simulink model "ConsoleSensor_harness"  (Simulink 7.7)
settings: Solver=FixedStepDiscrete  SolverMode=SingleTasking  StartTime=0.0  StopTime=100  FixedStep=0.01  RelTol=1e-3
InitFcn:
  | if signalbuilder('ConsoleSensor_harness/Signal_Builder','activegroup') == 4
  |   CD_CONSOLE_FUNCTION.DataType = 'uint8';
  |   CD_CONSOLE_FUNCTION.Value = 255;
  | else
  |   CD_CONSOLE_FUNCTION.DataType = 'uint8';
  |   CD_CONSOLE_FUNCTION.Value = 0;
  | end
undefined symbols (not defined in the file): ACTIVE, CD_CONSOLE_DEBOUNCE_ABSENT, CD_CONSOLE_DEBOUNCE_OORH, CD_CONSOLE_DEBOUNCE_OORL, CD_CONSOLE_DEBOUNCE_PRESENT, CD_CONSOLE_OORH, CD_CONSOLE_OORL, CD_CONSOLE_PRESENT_HIGH, CD_CONSOLE_PRESENT_LOW, INACTIVE, NON_FUNCTIONAL, NORMAL, OORH, OORL, sigbuilder_block, srate, SYS_NORMAL
libraries: MX_Library x2
settings Model: Creator=smindema  LastModifiedBy=aliebel  CovMetricSettings=dcm  CovForceBlockReductionOff=off  CovCumulativeReport=on  CovModelRefEnable=off
settings MATStruct: SampleTime=0.01  Offset=0  Priority=[1.0]
settings DataIOCC: LimitDataPoints=off  SaveOutput=off  SaveTime=off
settings OptimizationCC: BlockReduction=off  InlineParams=on  ExpressionFolding=off  StateBitsets=on  DataBitsets=on  UseTempVars=on  InitFltsAndDblsToZero=on  EfficientFloat2IntCast=on  OptimizeModelRefInitCode=on
settings DebuggingCC: SignalInfNanChecking=error  SignalRangeChecking=error  ReadBeforeWriteMsg=EnableAllAsError  WriteAfterWriteMsg=EnableAllAsError  WriteAfterReadMsg=EnableAllAsError  AlgebraicLoopMsg=error  ArtificialAlgebraicLoopMsg=error  SaveWithDisabledLinksMsg=error  SaveWithParameterizedLinksMsg=error  UnderspecifiedInitializationDetection=Simplified  BlockPriorityViolationMsg=error  SolverPrmCheckMsg=error  InheritedTsInSrcMsg=error  DiscreteInheritContinuousMsg=error  SigSpecEnsureSampleTimeMsg=error  CheckMatrixSingularityMsg=error  IntegerOverflowMsg=error  ParameterUnderflowMsg=error  ParameterPrecisionLossMsg=error  ParameterTunabilityLossMsg=error  UnderSpecifiedDataTypeMsg=error  UnnecessaryDatatypeConvMsg=warning  VectorMatrixConversionMsg=error  FcnCallInpInsideContextMsg=Enable All  SignalLabelMismatchMsg=error  UnconnectedInputMsg=error  UnconnectedOutputMsg=error  UnconnectedLineMsg=error  SFcnCompatibilityMsg=error  UniqueDataStoreMsg=error  BusObjectLabelMismatch=error  RootOutportRequireBusObject=error  AssertControl=DisableAll  ModelReferenceIOMsg=error  ModelReferenceIOMismatchMessage=error  ModelReferenceCSMismatchMessage=warning  UnknownTsInhSupMsg=error  ModelReferenceDataLoggingMessage=error  StrictBusMsg=ErrorOnBusTreatedAsVector
settings HardwareCC: ProdBitPerInt=16  ProdBitPerPointer=16  ProdIntDivRoundTo=Floor  ProdEndianess=BigEndian  ProdWordSize=16  ProdHWDeviceType=Motorola HC12
settings ModelReferenceCC: ModelReferenceNumInstancesAllowed=Single
settings SFSimCC: SimCustomHeaderCode="#include \"SendMsgNow.h\""  SimUserSources=SendMsgNow_Blank.c  SimUserIncludeDirs=functions
settings RTWCC: SystemTargetFile=ert.tlc  GenCodeOnly=on  TemplateMakefile=ert_default_tmf  Description=Real-Time Workshop Embedded Coder (no auto configuration)  GenerateReport=on  RetainRTWFile=on  ProcessScript=ert_make_rtw_hook  CustomInclude="\"C:\\Projects\\GEN IV\\GATEWAY\\Gtwy_256_Dev\\model\\functions\""  CustomSource=SendMsgNow.c  IncludeHyperlinkInReport=on  LaunchReport=on  IncludeERTFirstTime=on
settings RTWCC: CustomHeaderCode=|
  | #include "cpp_req_defines.h"
  | #include "hw_fin.h"
  | #include "cdata.h"
  | #include "SendMsgNow.h"
settings CodeAppCC: ForceParamTrailComments=on  IgnoreCustomStorageClasses=off  MangleLength=4  DefineNamingRule=UpperCase  ReqsInCode=on
settings ERTTargetCC: TargetFcnLib=ansi_tfl_tmw.mat  FunctionExecutionProfile=off  MultiwordLength=2048  IncludeMdlTerminateFcn=off  GeneratePreprocessorConditionals=Disable all  SuppressErrorStatus=on  SupportAbsoluteTime=off  SupportNonFinite=off  SupportComplex=off  PurelyIntegerCode=on  ParenthesesLevel=Maximum  ERTCustomFileTemplate=gen_rtw_req_defines_h.tlc  GlobalDataDefinition=InSeparateSourceFile  GlobalDataReference=InSeparateHeaderFile  PreserveExpressionOrder=on  PreserveIfCondition=on  ConvertIfToSwitch=off

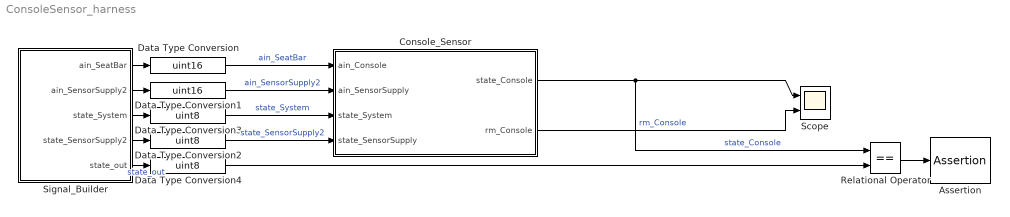
== system ConsoleSensor_harness ==
  Assertion : Assertion  Enabled=off
  Console_Sensor : Subsystem  TreatAsAtomicUnit=on  SystemSampleTime=srate  RTWFileName=mod_Inputs
      settings: RTWSystemCode=Function  RTWFcnNameOpts=Use subsystem name  RTWFileNameOpts=User specified
  Data Type Conversion : DataTypeConversion  OutDataTypeStr=uint16  RndMeth=Simplest
  Data Type Conversion1 : DataTypeConversion  OutDataTypeStr=uint16  RndMeth=Simplest
  Data Type Conversion2 : DataTypeConversion  OutDataTypeStr=uint8  RndMeth=Simplest
  Data Type Conversion3 : DataTypeConversion  OutDataTypeStr=uint8  RndMeth=Simplest
  Data Type Conversion4 : DataTypeConversion  OutDataTypeStr=uint8  RndMeth=Simplest
  Relational Operator : RelationalOperator  Operator===  OutDataTypeStr=boolean
  Scope : Scope  NumInputPorts=2
      settings: TimeRange=0.006402431848890444  YMin=15.52744536940686~200  YMax=16.93223204994796~1100  MaxDataPoints=50000
  Signal_Builder : Subsystem  Tag=STV Subsys  LoadFcn=sigbuilder_block('load',[202.5 82.5 1080 620.25 ]);  StartFcn=sigbuilder_block('start');  StopFcn=sigbuilder_block('stop');  ClipboardFcn=sigbuilder_block('clipboard');  mask(Sigbuilder block){}
      mask help: Sigbuilder GUI
      mask init:
      | if ~strcmp(get_param(bdroot(gcbh),'SimulationStatus'),'stopped') tuvar = sigbuilder_block('maskInit'); end
      settings: CopyFcn=sigbuilder_block('copy');  DeleteFcn=sigbuilder_block('delete');  ModelCloseFcn=sigbuilder_block('modelClose');  PreSaveFcn=sigbuilder_block('preSave');  NameChangeFcn=sigbuilder_block('namechange');  OpenFcn=sigbuilder_block('open',[202.5 82.5 1080 620.25 ]);  CloseFcn=sigbuilder_block('close');
      mask Display: plot(0,0,100,100,[10,10,40,40,10],[80,20,20,80,80],[40,10],[50,50], [40,27,10],[65,72,56],[40,25,25,10],[28,28,43,43]);
  wires:
  Console_Sensor/1(state_Console) -> Scope/1, Relational Operator/1  "state_Console"
  Signal_Builder/1(ain_SeatBar) -> Data Type Conversion/1
  Data Type Conversion/1 -> Console_Sensor/1(ain_Console)  "ain_SeatBar"
  Signal_Builder/2(ain_SensorSupply2) -> Data Type Conversion1/1
  Console_Sensor/2(rm_Console) -> Scope/2  "rm_Console"
  Relational Operator/1 -> Assertion/1
  Signal_Builder/5(state_out) -> Data Type Conversion4/1  "state_out"
  Data Type Conversion1/1 -> Console_Sensor/2(ain_SensorSupply)  "ain_SensorSupply2"
  Signal_Builder/4(state_SensorSupply2) -> Data Type Conversion2/1
  Data Type Conversion2/1 -> Console_Sensor/4(state_SensorSupply)  "state_SensorSupply2"
  Signal_Builder/3(state_System) -> Data Type Conversion3/1
  Data Type Conversion3/1 -> Console_Sensor/3(state_System)  "state_System"
  Data Type Conversion4/1 -> Relational Operator/2

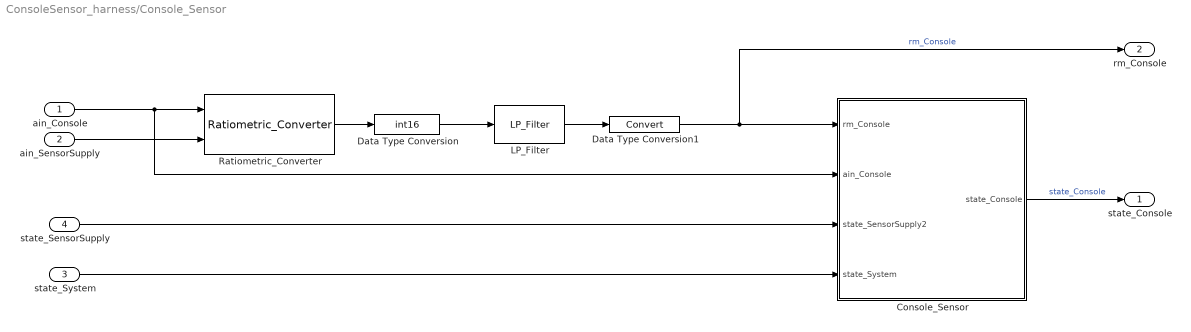
== system ConsoleSensor_harness/Console_Sensor ==
  ain_Console : Inport  OutDataTypeStr=uint16
  ain_SensorSupply : Inport  Port=2  OutDataTypeStr=uint16
  state_System : Inport  Port=3
  state_SensorSupply : Inport  Port=4
  Console_Sensor : Stateflow chart  TreatAsAtomicUnit=on
  Data Type Conversion : DataTypeConversion  OutDataTypeStr=int16  RndMeth=Zero
  Data Type Conversion1 : DataTypeConversion  RndMeth=Simplest
  LP_Filter : MX_Library/LP_Filter  SystemSampleTime=-1  GAIN=3
  Ratiometric_Converter : MX_Library/Ratiometric_Converter  SystemSampleTime=-1  multiplier=1000
  state_Console : Outport  OutDataTypeStr=uint8
  rm_Console : Outport  Port=2
  wires:
  Console_Sensor/1(state_Console) -> state_Console/1  "state_Console"
  ain_Console/1 -> Console_Sensor/2(ain_Console), Ratiometric_Converter/1
  Ratiometric_Converter/1 -> Data Type Conversion/1
  ain_SensorSupply/1 -> Ratiometric_Converter/2
  Data Type Conversion/1 -> LP_Filter/1
  LP_Filter/1 -> Data Type Conversion1/1
  Data Type Conversion1/1 -> Console_Sensor/1(rm_Console), rm_Console/1  "rm_Console"
  state_SensorSupply/1 -> Console_Sensor/3(state_SensorSupply2)
  state_System/1 -> Console_Sensor/4(state_System)

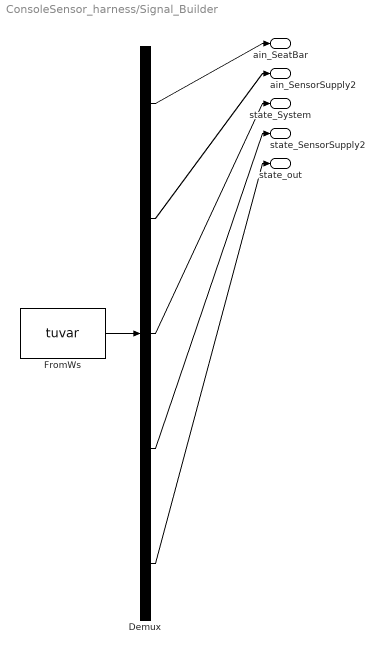
== system ConsoleSensor_harness/Signal_Builder ==
  Demux : Demux  Tag=STV Demux  Outputs=5
  FromWs : FromWorkspace  Tag=STV FromWs  VariableName=tuvar  SampleTime=0  SigBuilderData=DataTag0  VnvData=DataTag1
      SigBuilderData=|
      | common.afterFinalStr = 'Extrapolate'
      | common.sampleTime = 0
      | dataSet(1).timeRange = [0 100]
      | dataSet(1).name = 'OORL'
      | dataSet(2).timeRange = [0 100]
      | dataSet(2).name = 'OORH'
      | dataSet(3).timeRange = [0 100]
      | dataSet(3).name = 'Normal'
      | dataSet(4).timeRange = [0 100]
      | dataSet(4).name = 'NONFunctional'
      | sbobj.Groups(1).Name = 'OORL'
      | sbobj.Groups(1).Signals(1).Name = 'ain_SeatBar'
      | sbobj.Groups(1).Signals(1).XData = [0 2 2 2.03 2.03 8.4 8.4 8.5 8.5 10.02 10.02 20.4 20.4 40 40 40.03 40.03 44.2 44.2 52 52 52.04 52.04 60.2 60.2 60.41 60.41 60.43 60.43 70 70 85.8 85.8 89.8 89.8 96.8 96.8 100]
      | sbobj.Groups(1).Signals(1).YData = [200 200 0 0 200 200 0 0 200 200 0 0 200 200 620 620 200 200 0 0 200 200 0 0 200 200 600 600 200 200 600 600 200 200 100 100 210 210]
      | sbobj.Groups(1).Signals(2).Name = 'ain_SensorSupply2'
      | sbobj.Groups(1).Signals(2).XData = [0 100]
      | sbobj.Groups(1).Signals(2).YData = [850 850]
      | sbobj.Groups(1).Signals(3).Name = 'state_System'
      | sbobj.Groups(1).Signals(3).XData = [0 27.5 27.5 31.6 31.6 100]
      | sbobj.Groups(1).Signals(3).YData = [1 1 0 0 1 1]
      | sbobj.Groups(1).Signals(4).Name = 'state_SensorSupply2'
      | sbobj.Groups(1).Signals(4).XData = [0 100]
      | sbobj.Groups(1).Signals(4).YData = [8 8]
      | sbobj.Groups(1).Signals(5).Name = 'state_out'
      | sbobj.Groups(1).Signals(5).XData = [0 0.22 0.22 8.45 8.45 27.5 27.5 31.81 31.81 44.25 44.25 100]
      | sbobj.Groups(1).Signals(5).YData = [255 255 0 0 22 22 255 255 0 0 22 22]
      | sbobj.Groups(2).Name = 'OORH'
      | sbobj.Groups(2).Signals(1).Name = 'ain_SeatBar'
      | sbobj.Groups(2).Signals(1).XData = [0 2 40 40 40.01 40.01 44.2 44.2 52 52 52.04 52.04 60.2 60.2 60.41 60.41 60.43 60.43 100]
      | sbobj.Groups(2).Signals(1).YData = [600 600 600 900 900 600 600 900 900 200 200 900 900 200 200 600 600 195 210]
      | sbobj.Groups(2).Signals(2).Name = 'ain_SensorSupply2'
      | sbobj.Groups(2).Signals(2).XData = [0 100]
      | sbobj.Groups(2).Signals(2).YData = [850 850]
      | sbobj.Groups(2).Signals(3).Name = 'state_System'
      | sbobj.Groups(2).Signals(3).XData = [0 72.4 72.4 74.8 74.8 100]
      | sbobj.Groups(2).Signals(3).YData = [1 1 0 0 1 1]
      | sbobj.Groups(2).Signals(4).Name = 'state_SensorSupply2'
      | sbobj.Groups(2).Signals(4).XData = [0 100]
      | sbobj.Groups(2).Signals(4).YData = [8 8]
      | sbobj.Groups(2).Signals(5).Name = 'state_out'
      | sbobj.Groups(2).Signals(5).XData = [0 0.22 0.22 44.25 44.25 72.4 72.4 75.01 75.01 100]
      | sbobj.Groups(2).Signals(5).YData = [255 255 0 0 21 21 255 255 0 0]
      | sbobj.Groups(3).Name = 'Normal'
      | sbobj.Groups(3).Signals(1).Name = 'ain_SeatBar'
      | sbobj.Groups(3).Signals(1).XData = [0 10 10 10.04 10.04 20 20 20.1 20.1 20.11 20.11 32 32 32.1 32.1 40 40 40.02 40.02 40.04 40.04 46.7 46.7 46.8 46.8 69.8 69.8 90.1 90.1 100]
      | sbobj.Groups(3).Signals(1).YData = [390 390 500 500 395 395 498 498 200 200 498 498 98 98 498 498 200 200 500 500 405 405 135 135 405 405 96 96 400 400]
      | sbobj.Groups(3).Signals(2).Name = 'ain_SensorSupply2'
      | sbobj.Groups(3).Signals(2).XData = [0 100]
      | sbobj.Groups(3).Signals(2).YData = [850 850]
      | sbobj.Groups(3).Signals(3).Name = 'state_System'
      | sbobj.Groups(3).Signals(3).XData = [0 53 53 56.2 56.2 100]
      | sbobj.Groups(3).Signals(3).YData = [1 1 0 0 1 1]
      | sbobj.Groups(3).Signals(4).Name = 'state_SensorSupply2'
      | sbobj.Groups(3).Signals(4).XData = [0 61.4 61.4 65 65 100]
      | sbobj.Groups(3).Signals(4).YData = [8 8 4 4 8 8]
      | sbobj.Groups(3).Signals(5).Name = 'state_out'
      | sbobj.Groups(3).Signals(5).XData = [0 0.07 0.07 20.32 20.32 32.18 32.18 32.43 32.43 40.1 40.1 53 53 56.26 56.26 61.62 61.62 65.05 65.05 70.03 70.03 90.24 90.24 100]
      | sbobj.Groups(3).Signals(5).YData = [255 255 1 1 0 0 1 1 0 0 1 1 255 255 1 1 0 0 1 1 0 0 1 1]
      | sbobj.Groups(4).Name = 'NONFunctional'
      | sbobj.Groups(4).Signals(1).Name = 'ain_SeatBar'
      | sbobj.Groups(4).Signals(1).XData = [0 10 10 10.04 10.04 20 20 20.1 20.1 20.11 20.11 32 32 32.1 32.1 40 40 40.02 40.02 40.04 40.04 69.8 69.8 90.1 90.1 100]
      | sbobj.Groups(4).Signals(1).YData = [200 200 500 500 200 200 498 498 200 200 498 498 98 98 498 498 200 200 500 500 200 200 96 96 200 200]
      | sbobj.Groups(4).Signals(2).Name = 'ain_SensorSupply2'
      | sbobj.Groups(4).Signals(2).XData = [0 100]
      | sbobj.Groups(4).Signals(2).YData = [850 850]
      | sbobj.Groups(4).Signals(3).Name = 'state_System'
      | sbobj.Groups(4).Signals(3).XData = [0 100]
      | sbobj.Groups(4).Signals(3).YData = [1 1]
      | sbobj.Groups(4).Signals(4).Name = 'state_SensorSupply2'
      | sbobj.Groups(4).Signals(4).XData = [0 100]
      | sbobj.Groups(4).Signals(4).YData = [8 8]
      | sbobj.Groups(4).Signals(5).Name = 'state_out'
      | sbobj.Groups(4).Signals(5).XData = [0 100]
      | sbobj.Groups(4).Signals(5).YData = [255 255]
  ain_SeatBar : Outport  Tag=STV Outport
  ain_SensorSupply2 : Outport  Tag=STV Outport  Port=2
  state_System : Outport  Tag=STV Outport  Port=3
  state_SensorSupply2 : Outport  Tag=STV Outport  Port=4
  state_out : Outport  Tag=STV Outport  Port=5
  wires:
  FromWs/1 -> Demux/1
  Demux/1 -> ain_SeatBar/1
  Demux/2 -> ain_SensorSupply2/1
  Demux/3 -> state_System/1
  Demux/4 -> state_SensorSupply2/1
  Demux/5 -> state_out/1

== stateflow chart Console_Sensor/Console_Sensor ==
  state NON_FUNCTIONAL
    en:
    state_Console = NON_FUNCTIONAL;
  state STATE
    state NORMAL
      state ABSENT
        state ABSENT
          en:
          state_Console = INACTIVE;
          %SendMsg_BICSControl_Now();
        state DEBOUNCE_ABSENT
          en:
          debounceCount = 0;
          du:
          debounceCount++;
        (default) -> DEBOUNCE_ABSENT
        DEBOUNCE_ABSENT -> STATE.NORMAL.ABSENT.ABSENT : [(debounceCount >= CD_CONSOLE_DEBOUNCE_ABSENT)...
            | || (state_Console == INACTIVE)]
      state PRESENT
        state PRESENT
          en:
          state_Console = ACTIVE;
          %SendMsg_BICSControl_Now();
        state DEBOUNCE_PRESENT
          en:
          debounceCount = 0;
          du:
          debounceCount++;
        DEBOUNCE_PRESENT -> STATE.NORMAL.PRESENT.PRESENT : [(debounceCount >= CD_CONSOLE_DEBOUNCE_PRESENT)...
            | || (state_Console == ACTIVE)]
        (default) -> DEBOUNCE_PRESENT
      STATE.NORMAL.ABSENT -> STATE.NORMAL.PRESENT : [(rm_Console >= CD_CONSOLE_PRESENT_LOW) ...
          | && (rm_Console <= CD_CONSOLE_PRESENT_HIGH)...
          | && (state_SensorSupply2 == NORMAL)]
      STATE.NORMAL.PRESENT -> STATE.NORMAL.ABSENT : [(rm_Console < CD_CONSOLE_PRESENT_LOW)...
          | || (rm_Console > CD_CONSOLE_PRESENT_HIGH)...
          | || (state_SensorSupply2 != NORMAL)]
      (default) -> STATE.NORMAL.ABSENT
    state OORH
      state DEBOUNCE
        en:
        debounceCount = 0;
        du:
        debounceCount++;
      state OORH
        en:
        state_Console = OORH;
        %SendMsg_BICSControl_Now();
      STATE.OORH.DEBOUNCE -> STATE.OORH.OORH : [(debounceCount >= CD_CONSOLE_DEBOUNCE_OORH)]
      (default) -> STATE.OORH.DEBOUNCE
    state OORL
      state DEBOUNCE
        en:
        debounceCount = 0;
        du:
        debounceCount++;
      state OORL
        en:
        state_Console = OORL;
        %SendMsg_BICSControl_Now();
      (default) -> STATE.OORL.DEBOUNCE
      STATE.OORL.DEBOUNCE -> STATE.OORL.OORL : [(debounceCount >= CD_CONSOLE_DEBOUNCE_OORL)]
    NORMAL -> STATE.OORH [order 2] : [(ain_Console >= CD_CONSOLE_OORH)]
    NORMAL -> STATE.OORL [order 1] : [(ain_Console <= CD_CONSOLE_OORL)]
    (default) -> NORMAL
    STATE.OORH -> NORMAL : [(ain_Console< CD_CONSOLE_OORH)...
        | && (state_Console != OORH)]
    STATE.OORL -> NORMAL : [(ain_Console > CD_CONSOLE_OORL)...
        | && (state_Console != OORL)]
  (default) -> NON_FUNCTIONAL
  NON_FUNCTIONAL -> STATE : [(CD_CONSOLE_FUNCTION != NON_FUNCTIONAL)...
      | && (state_System == SYS_NORMAL)]
  STATE -> NON_FUNCTIONAL : [(state_System != SYS_NORMAL)]
  data: state_Console output uint8; rm_Console input uint16; CD_CONSOLE_PRESENT_LOW parameter uint16; CD_CONSOLE_PRESENT_HIGH parameter uint16; CD_CONSOLE_FUNCTION parameter uint8; CD_CONSOLE_DEBOUNCE_PRESENT parameter uint16; CD_CONSOLE_DEBOUNCE_ABSENT parameter uint16; debounceCount local uint16 =0; CD_CONSOLE_OORH parameter uint16; CD_CONSOLE_DEBOUNCE_OORH parameter uint16; CD_CONSOLE_OORL parameter uint16; CD_CONSOLE_DEBOUNCE_OORL parameter uint16; ain_Console input uint16; ACTIVE parameter uint8 =1; INACTIVE parameter uint8 =0; OORH parameter uint8 =21; OORL parameter uint8 =22; NON_FUNCTIONAL parameter uint8 =255; state_SensorSupply2 input uint8; NORMAL parameter uint8; state_System input uint8; SYS_NORMAL parameter uint8
  data rm_Console settings: description=Ratiometric value of the seatbar, calculated based on the sensor supply voltage and the analog voltage.
